simulink model "project"  (R2018b)
settings: Solver=ode3  StartTime=0.0  StopTime=10  RelTol=1e-3  EnableMultiTasking=on
libraries: legoev3lib x10
settings Model: FPTRunName=Active  ExtModeTrigDuration=2  Creator=jloehnertz  LastModifiedBy=jloehnertz
settings SolverCC: PositivePriorityOrder=on
settings DataIOCC: LimitDataPoints=on  SaveFormat=Array
settings OptimizationCC: ExpressionDepthLimit=2147483647  LifeSpan=Inf  MaxStackSize=64
settings DebuggingCC: UnderspecifiedInitializationDetection=Classic  MergeDetectMultiDrivingBlocksExec=none  FcnCallInpInsideContextMsg=warning  AllowSymbolicDim=off  StateNameClashWarn=warning  SFUnexpectedBacktrackingDiag=warning  SFNoUnconditionalDefaultTransitionDiag=warning  SFExecutionAtInitializationDiag=none
settings HardwareCC: ProdBitPerPointer=32  ProdBitPerSizeT=32  ProdBitPerPtrDiffT=32  ProdLargestAtomicInteger=Long  ProdWordSize=32  ProdHWDeviceType=ARM Compatible->ARM 9  UseEmbeddedCoderFeatures=off  UseSimulinkCoderFeatures=off
settings ModelReferenceCC: PropagateSignalLabelsOutOfModel=off
settings SFSimCC: SimUseLocalCustomCode=off
settings RTWCC: SystemTargetFile=ert.tlc  HardwareBoard=LEGO MINDSTORMS EV3  TemplateMakefile=ert_default_tmf  GenerateReport=on  RTWVerbose=off  RTWUseLocalCustomCode=off  Toolchain=Sourcery G++ Lite v2009q3  BuildConfiguration=Faster Runs  LaunchReport=on
settings CodeAppCC: ForceParamTrailComments=on  OperatorAnnotations=on  StateflowObjectComments=on  MATLABSourceComments=on
settings ERTTargetCC: MultiwordLength=2048  ERTCustomFileBanners=off  SupportContinuousTime=on  SupportNonInlinedSFcns=on  RemoveResetFunc=off  SupportVariableSizeSignals=on  ModelStepFunctionPrototypeControlCompliant=off
settings ConfigComp: CovMetricSettings=dw  CovHtmlReporting=on  CovSaveCumulativeToWorkspaceVar=on  CovSaveSingleToWorkspaceVar=on  CovExternalEMLEnable=off  CovSFcnEnable=off

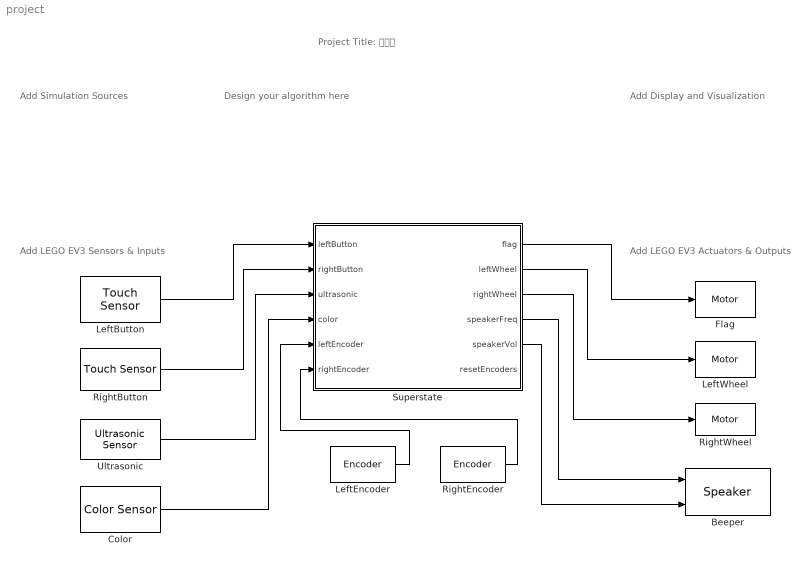
== system project ==
  note: Project Title: 🔮🐙🏝️
  note: Add LEGO EV3 Sensors & Inputs
  note: Add LEGO EV3 Actuators & Outputs
  note: Add Display and Visualization
  note: Design your algorithm here
  note: Add Simulation Sources
  Beeper : legoev3lib/Speaker  sinputMode=Frequency and volume  sspeakerFreq=100  sspeakerVolume=50  sspeakerDuration=100
      settings: SourceProductName=Simulink Support Package for LEGO MINDSTORMS EV3 Hardware  SourceProductBaseCode=LEGOEV3
  Color : legoev3lib/Color Sensor  portNumber=3  mode=Color  sampleTime=0.1
      settings: SourceProductName=Simulink Support Package for LEGO MINDSTORMS EV3 Hardware  SourceProductBaseCode=LEGOEV3
  Flag : legoev3lib/Motor  sportNumber=A  sstopAction=Brake
  LeftButton : legoev3lib/Touch Sensor  portNumber=1  sampleTime=0.1
      settings: SourceProductName=Simulink Support Package for LEGO MINDSTORMS EV3 Hardware  SourceProductBaseCode=LEGOEV3
  LeftEncoder : legoev3lib/Encoder  portNumber=C  opMode=Reset by external signal  sampleTime=0.1
      settings: SourceProductName=Simulink Support Package for LEGO MINDSTORMS EV3 Hardware  SourceProductBaseCode=LEGOEV3
  LeftWheel : legoev3lib/Motor  sportNumber=C  sstopAction=Brake
  RightButton : legoev3lib/Touch Sensor  portNumber=2  sampleTime=0.1
      settings: SourceProductName=Simulink Support Package for LEGO MINDSTORMS EV3 Hardware  SourceProductBaseCode=LEGOEV3
  RightEncoder : legoev3lib/Encoder  portNumber=B  opMode=Reset by external signal  sampleTime=0.1
      settings: SourceProductName=Simulink Support Package for LEGO MINDSTORMS EV3 Hardware  SourceProductBaseCode=LEGOEV3
  RightWheel : legoev3lib/Motor  sportNumber=B  sstopAction=Brake
  Superstate : Stateflow chart  TreatAsAtomicUnit=on
  Ultrasonic : legoev3lib/Ultrasonic Sensor  PortNumber=4  sampleTime=0.1
      settings: SourceProductName=Simulink Support Package for LEGO MINDSTORMS EV3 Hardware  SourceProductBaseCode=LEGOEV3
  wires:
  LeftButton/1 -> Superstate/1(leftButton)
  RightButton/1 -> Superstate/2(rightButton)
  Superstate/1(flag) -> Flag/1
  Superstate/3(rightWheel) -> RightWheel/1
  Superstate/2(leftWheel) -> LeftWheel/1
  Superstate/4(speakerFreq) -> Beeper/1
  Superstate/5(speakerVol) -> Beeper/2
  Ultrasonic/1 -> Superstate/3(ultrasonic)
  Color/1 -> Superstate/4(color)
  RightEncoder/1 -> Superstate/6(rightEncoder)
  LeftEncoder/1 -> Superstate/5(leftEncoder)

== stateflow chart project/Superstate ==
  state Manual1
    state RESET
    state AUTONOMOUS
      entry:
      send(startAutonomous)
    state TURNLEFT
      entry:
      leftWheel = -scanSpeed;
      rightWheel = scanSpeed;
    state MANUAL
      entry:
      leftWheel = 0;
      rightWheel = 0;
    state HOLD
    state WAIT
    state STOP
    state FORWARD
      entry:
      leftWheel = 30;
      rightWheel = 30;
    state SIDEMISSION
      entry:
      send(startSidemission)
    state TURNRIGHT
      entry:
      leftWheel = scanSpeed;
      rightWheel = -scanSpeed;
    RESET -> MANUAL [order 1] : after(1, sec)
    RESET -> AUTONOMOUS [order 2] : [not(leftButton == 1 & rightButton == 1)]
    TURNLEFT -> MANUAL : [not(leftButton == 1 & rightButton == 0)]
    MANUAL -> TURNLEFT [order 1] : [leftButton == 1 & rightButton == 0]
    WAIT -> AUTONOMOUS [order 2] : [not(leftButton == 1 & rightButton == 1)]
    (default) -> MANUAL
    HOLD -> WAIT [order 2] : after(1, sec)
    MANUAL -> HOLD [order 3] : [leftButton == 1 & rightButton == 1]
    HOLD -> FORWARD [order 1] : [not(leftButton == 1 & rightButton == 1)]
    WAIT -> SIDEMISSION [order 1] : after(2, sec)
    STOP -> MANUAL : [leftButton == 0 & rightButton == 0]
    FORWARD -> STOP : [not(leftButton == 0 & rightButton == 0)]
    MANUAL -> TURNRIGHT [order 2] : [leftButton == 0 & rightButton == 1]
    TURNRIGHT -> MANUAL : [not(leftButton == 0 & rightButton == 1)]
  state Autonomous
    state Approach
      state Start
        entry:
        leftWheel = 20;
        rightWheel = 20;
      state Wait
        entry:
        leftWheel = 0;
        rightWheel = 0;
      state Exit
        entry:
        send(startFlee)
      (default) -> Start
      Start -> Wait : [ultrasonic < stopDistance]
      Wait -> Exit : after(5, sec)
    state Flee1
      state Beep1
        entry:
        speakerFreq = 600;
        speakerVol = desiredSpeakerVol;
      state ResetEncoders
        entry:
        resetEncoders = 1;
        exit:
        resetEncoders = 0;
      state Turn
        entry:
        speakerFreq = 0;
        speakerVol = 0;
        leftWheel = driveSpeed;
        rightWheel = -driveSpeed;
      state MoveForward
        entry:
        leftWheel = driveSpeed;
        rightWheel = driveSpeed;
      state BeepStop
        entry:
        speakerFreq = 0;
        speakerVol = 0;
        send(initLineFollow)
      state Beep
        entry:
        speakerFreq = 600;
        speakerVol = desiredSpeakerVol;
      state StopRobot
        entry:
        leftWheel = 0;
        rightWheel = 0;
      (default) -> Autonomous.Flee1.ResetEncoders
      Turn -> MoveForward : [leftEncoder - rightEncoder > 3 * 90]
      Beep1 -> Turn : after(0.5, sec)
      MoveForward -> StopRobot : after(0.5, sec)[color == 1]
      Autonomous.Flee1.ResetEncoders -> Beep1 : after(0.1,sec)
      StopRobot -> Beep
      Beep -> BeepStop : after(0.5, sec)
    state Flee2
      state Init
        entry:
        leftWheel = 0;
        rightWheel = 0;
      state Maneuver
        state TryLeft
          entry:
          lastDirection = 0;
          waitTime = waitTime * 2;
          state LeftCheck
            entry:
            leftWheel = -scanSpeed;
            rightWheel = scanSpeed / 2;
          state ALittleRight
            entry:
            leftWheel = scanSpeed;
            rightWheel = -scanSpeed / 2;
          state WaitForWhite
          (default) -> LeftCheck
          Autonomous.Flee2.Maneuver.TryLeft.WaitForWhite -> ALittleRight : [color ~= 1]
          LeftCheck -> Autonomous.Flee2.Maneuver.TryLeft.WaitForWhite [order 2] : [color == 1]
        state Follow
          entry:
          leftWheel = driveSpeed;
          rightWheel = driveSpeed;
        state LastDirectionDecision
          entry: waitTime = 0.1;
        state TryRight
          entry:
          lastDirection = 1;
          waitTime = waitTime * 2;
          state ALittleLeft
            entry:
            leftWheel = -scanSpeed;
            rightWheel = scanSpeed / 2;
          state WaitForWhite
          state RightCheck
            entry:
            leftWheel = scanSpeed;
            rightWheel = -scanSpeed / 2;
          (default) -> RightCheck
          Autonomous.Flee2.Maneuver.TryRight.WaitForWhite -> ALittleLeft : [color ~= 1]
          RightCheck -> Autonomous.Flee2.Maneuver.TryRight.WaitForWhite [order 2] : [color == 1]
        state Stop
          entry:
          leftWheel = 0;
          rightWheel = 0;
        (default) -> Follow
        LastDirectionDecision -> TryLeft [order 1] : [lastDirection == 0]
        Autonomous.Flee2.Maneuver.Stop -> Follow [order 3] : [color == 1]
        Follow -> Autonomous.Flee2.Maneuver.Stop : [color ~= 1]
        LeftCheck -> TryRight [order 1] : after(waitTime, sec)[color ~= 1]
        ALittleRight -> Autonomous.Flee2.Maneuver.Stop : [color == 1]
        RightCheck -> TryLeft [order 1] : after(waitTime, sec)[color ~= 1]
        LastDirectionDecision -> TryRight [order 2] : [lastDirection == 1]
        Autonomous.Flee2.Maneuver.Stop -> LastDirectionDecision [order 2] : [color ~= 1]
        ALittleLeft -> Autonomous.Flee2.Maneuver.Stop : [color == 1]
      state RaiseFlagAndBeep
        state BeepAndRaiseFlag
          entry:
          speakerFreq = 600;
          speakerVol = desiredSpeakerVol;
          flag = 1;
        state StopBeeping
          entry:
          speakerVol = 0;
        (default) -> BeepAndRaiseFlag
        BeepAndRaiseFlag -> StopBeeping : after(0.5, sec)
      (default) -> Init
      Init -> Maneuver : [color == 1]
      Autonomous.Flee2.Maneuver.Stop -> RaiseFlagAndBeep [order 1] : [color == 2]
    state InitLineFollow
      state ChooseDirection
      state TurnLeft
        entry:
        leftWheel = -scanSpeed;
        rightWheel = 0;
      state TurnRight
        entry:
        leftWheel = scanSpeed;
        rightWheel = -scanSpeed / 2;
      state Stop
        entry:
        leftWheel = 0;
        rightWheel = 0;
        send(startLineFollow);
      (default) -> ChooseDirection
      ChooseDirection -> TurnLeft [order 1] : [turnDirectionAfterFleeing == 0]
      ChooseDirection -> TurnRight [order 2] : [turnDirectionAfterFleeing == 1]
      TurnLeft -> Autonomous.InitLineFollow.Stop : after(0.5, sec)
      TurnRight -> Autonomous.InitLineFollow.Stop : after(0.5, sec)
    (default) -> Approach
    Approach -> Flee1 : [startFlee]
    Flee1 -> InitLineFollow : [initLineFollow]
    InitLineFollow -> Flee2 : [startLineFollow]
  state Sidemission
    state Do360NoScope
      entry:
      distanceNearestObstacle = 100;
      startRotation = rightEncoder - leftEncoder;
      speakerFreq = 0;
      speakerVol = 0;
      leftWheel = -scanSpeed;
      rightWheel = scanSpeed;
      state UpdateNearestObstacle
        entry:
        distanceNearestObstacle = ultrasonic;
        rotationNearestObstacle = rightEncoder - leftEncoder;
      state ResetEncoders
        entry:
        resetEncoders = 1;
        exit:
        resetEncoders = 0;
      state SearchNearestObstacle
      state StopSearch
        entry:
        leftWheel = 0;
        rightWheel = 0;
      state ReturnToNearestObstacle
        entry:
        leftWheel = scanSpeed;
        rightWheel = -scanSpeed;
      state StopReturnAndBeep
        entry:
        leftWheel = 0;
        rightWheel = 0;
        speakerFreq = 600;
        speakerVol = 55;
      state BeepRealQuick
        entry:
        speakerFreq = 600;
        speakerVol = 55;
        flag = scanSpeed;
      state StopApproaching
        entry:
        leftWheel = 0;
        rightWheel = 0;
      state StopBeepAndApproach
        entry:
        speakerFreq = 0;
        speakerVol = 0;
        leftWheel = 20;
        rightWheel = 20;
      state StopFlag
        entry:
        flag = 0;
        send(endSidemission);
      state ReverseFlag
        entry:
        speakerFreq = 0;
        speakerVol = 0;
        flag = -scanSpeed;
      (default) -> Sidemission.Do360NoScope.ResetEncoders
      SearchNearestObstacle -> UpdateNearestObstacle [order 1] : [ultrasonic < distanceNearestObstacle]
      Sidemission.Do360NoScope.ResetEncoders -> SearchNearestObstacle : after(0.1, sec)
      UpdateNearestObstacle -> SearchNearestObstacle
      SearchNearestObstacle -> StopSearch [order 2] : [rightEncoder - leftEncoder + startRotation >= 4 * 360]
      ReturnToNearestObstacle -> StopReturnAndBeep : [rightEncoder - leftEncoder <= rotationNearestObstacle]
      StopSearch -> ReturnToNearestObstacle
      StopReturnAndBeep -> StopBeepAndApproach : after(0.5, sec)
      StopApproaching -> BeepRealQuick
      StopBeepAndApproach -> StopApproaching : [ultrasonic < 21]
      BeepRealQuick -> ReverseFlag : after(2, sec)
      ReverseFlag -> StopFlag : after(2, sec)
    (default) -> Do360NoScope
  (default) -> Manual1
  Autonomous -> RESET : [leftButton == 1 & rightButton == 1]
  Manual1 -> (history) [order 1] : [startAutonomous]
  Manual1 -> Sidemission [order 2] : [startSidemission]
  Sidemission -> Manual1 : [endSidemission]
  data: leftButton input; rightButton input; flag output =0; leftWheel output; rightWheel output; speakerFreq output; speakerVol output; ultrasonic input; color input; stopDistance constant double =15; resetEncoders output; leftEncoder input; rightEncoder input; driveSpeed constant double =50; lastDirection local =0; scanSpeed constant double =25; waitTime local; desiredSpeakerVol constant double =55; turnDirectionAfterFleeing local =0; startRotation local; rotationNearestObstacle local; distanceNearestObstacle local
  events: startFlee local FUNCTION_CALL_EVENT; startAutonomous local FUNCTION_CALL_EVENT; initLineFollow local FUNCTION_CALL_EVENT; startLineFollow local FUNCTION_CALL_EVENT; endSidemission local FUNCTION_CALL_EVENT; startSidemission local FUNCTION_CALL_EVENT
